simulink model "adaptive_dcmotor_2nd_hw"  (R2025b)
settings: Solver=FixedStepAuto  StartTime=0.0  StopTime=inf  FixedStep=0.08  RelTol=1e-3  EnableMultiTasking=on
libraries: arduinolib x3, arduinosensorlib x1
settings Model: Creator=Lenard  LastModifiedBy=Felix
settings SolverCC: AutoInsertRateTranBlk=on
settings OptimizationCC: EnhancedBackFolding=on  PassReuseOutputArgsAs=Individual arguments  ZeroExternalMemoryAtStartup=off  ZeroInternalMemoryAtStartup=off  MaxStackSize=64  OptimizeBlockOrder=speed  DifferentSizesBufferReuse=on  OptimizationCustomize=off  EfficientTunableParamExpr=on
settings DebuggingCC: ParameterTunabilityLossMsg=error
settings HardwareCC: ProdBitPerPointer=32.0  ProdBitPerSizeT=32.0  ProdBitPerPtrDiffT=32.0  ProdLargestAtomicInteger=Long  ProdLargestAtomicFloat=Double  ProdWordSize=32.0  ProdHWDeviceType=ARM Compatible->ARM Cortex
settings SFSimCC: MATLABDynamicMemAlloc=off
settings RTWCC: SystemTargetFile=ert.tlc  HardwareBoard=ESP32-WROOM (Arduino Compatible)  TLCOptions="-aInlineSetEventsForThisBaseRateFcn=TLC_FALSE -aSuppressMultiTaskScheduler=TLC_FALSE  -aRateBasedStepFcn=0"  TemplateMakefile=ert_default_tmf  Toolchain=ESP32  BuildConfiguration=Faster Runs  Description=Embedded Coder
settings CodeAppCC: ForceParamTrailComments=on  IgnoreCustomStorageClasses=off  OperatorAnnotations=on  SimulinkDataObjDesc=on  SFDataObjDesc=on  InsertBlockDesc=on
settings ERTTargetCC: ExtModeTransport=3.0  ExtModeStaticAlloc=on  ExtModeAutomaticAllocSize=off  ExtModeStaticAllocSize=65536.0  ExtModeMexFile=ext_xcp  ExtModeIntrfLevel=Level2 - Open  InlinedParameterPlacement=Hierarchical  SupportContinuousTime=on  SupportVariableSizeSignals=on

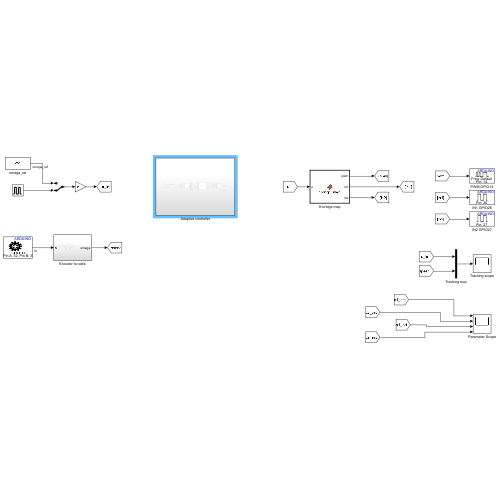
[thumbnail: Simulink's stored preview of the top-level diagram]
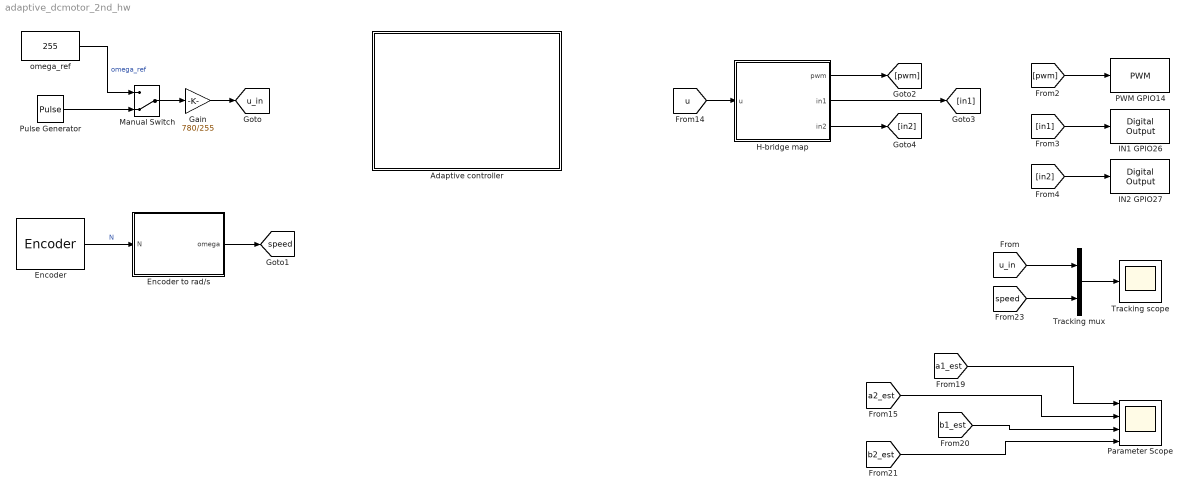
== system adaptive_dcmotor_2nd_hw ==
  Adaptive controller : Subsystem
  Encoder : arduinosensorlib/Encoder  InputA=32  InputB=33  Mode=No reset  SampleTime=0.08
  Encoder to rad/s : Subsystem
  Gain : Gain  Gain=780/255
  H-bridge map : MATLAB Function  TreatAsAtomicUnit=on
  IN1 GPIO26 : arduinolib/Digital Output  pinNumber=26  Direction=output  blockPlatform=arduino
  IN2 GPIO27 : arduinolib/Digital Output  pinNumber=27  Direction=output  blockPlatform=arduino
  Manual Switch : ManualSwitch  CurrentSetting=0
  PWM GPIO14 : arduinolib/PWM  pinNumber=14  frequencyType=Default  desiredFrequency=490.2  achievableFrequency=490.2
  Parameter Scope : Scope  NumInputPorts=4
      settings: ActiveDisplayYMinimum=-1590.0375907934126  ActiveDisplayYMaximum=2454.7527089363357
  Pulse Generator : DiscretePulseGenerator  PulseType=Time based  Amplitude=255  Period=8  PulseWidth=50  VectorParams1D=off
  Tracking mux : Mux  Inputs=2
  Tracking scope : Scope
      settings: ActiveDisplayYMinimum=-11603.301483749512  ActiveDisplayYMaximum=9185.7875106822521  DataLoggingVariableName=step
  omega_ref : Constant  Value=255  SampleTime=0.08
  tag scope: speed=global, u_in=global
  wires:
  Encoder/1 -> Encoder to rad/s/1(N)  "N"
  Pulse Generator/1 -> Manual Switch/2
  Gain/1 -> [u_in]
  Manual Switch/1 -> Gain/1
  omega_ref/1 -> Manual Switch/1  "omega_ref"
  Encoder to rad/s/1(omega) -> [speed]
  [pwm] -> PWM GPIO14/1
  [in1] -> IN1 GPIO26/1
  [in2] -> IN2 GPIO27/1
  H-bridge map/1(pwm) -> [pwm]
  H-bridge map/2(in1) -> [in1]
  H-bridge map/3(in2) -> [in2]
  [u] -> H-bridge map/1(u)
  Tracking mux/1 -> Tracking scope/1
  [u_in] -> Tracking mux/1
  [speed] -> Tracking mux/2
  [a2_est] -> Parameter Scope/2
  [b2_est] -> Parameter Scope/4
  [a1_est] -> Parameter Scope/1
  [b1_est] -> Parameter Scope/3

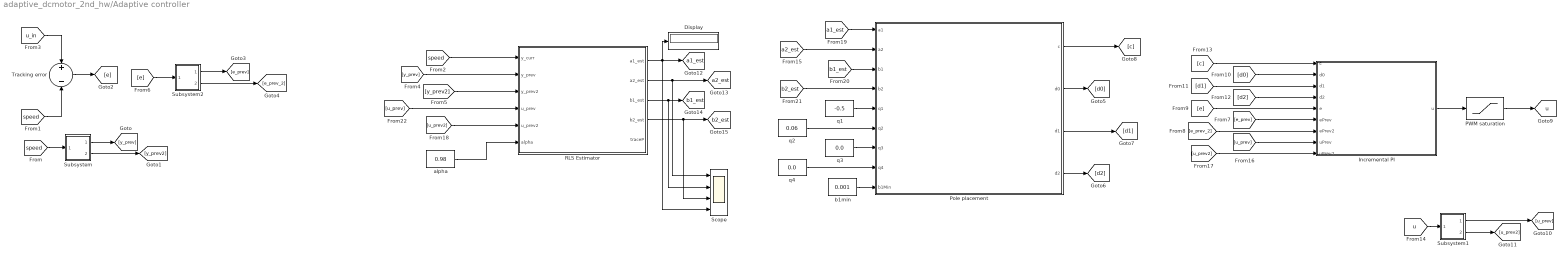
== system adaptive_dcmotor_2nd_hw/Adaptive controller ==
  Display : Display
  Incremental PI : MATLAB Function  TreatAsAtomicUnit=on
  PWM saturation : Saturate  UpperLimit=255  LowerLimit=0
  Pole placement : MATLAB Function  TreatAsAtomicUnit=on
  RLS Estimator : MATLAB Function  TreatAsAtomicUnit=on
  Scope : Scope  NumInputPorts=4
      settings: ActiveDisplayYMinimum=-1.9835538940406421  ActiveDisplayYMaximum=2.3467419345122842  DataLoggingVariableName=param
  Subsystem : Subsystem
  Subsystem1 : Subsystem
  Subsystem2 : Subsystem
  Tracking error : Sum  Inputs=+-
  alpha : Constant  Value=0.98
  b1min : Constant  Value=0.001
  q1 : Constant  Value=-0.5
  q2 : Constant  Value=0.06
  q3 : Constant  Value=0.0
  q4 : Constant  Value=0.0
  tag scope: a1_est=global, a2_est=global, b1_est=global, b2_est=global, u=global
  wires:
  alpha/1 -> RLS Estimator/6(alpha)
  Incremental PI/1(u) -> PWM saturation/1
  PWM saturation/1 -> [u]
  Pole placement/1(c) -> [c]
  q1/1 -> Pole placement/5(q1)
  q2/1 -> Pole placement/6(q2)
  q3/1 -> Pole placement/7(q3)
  q4/1 -> Pole placement/8(q4)
  b1min/1 -> Pole placement/9(b1Min)
  Subsystem1/1(Out1) -> [u_prev]
  Subsystem1/2(Out2) -> [u_prev2]
  [speed] -> Tracking error/2
  [speed] -> RLS Estimator/1(y_curr)
  [speed] -> Subsystem/1(In1)
  [u_in] -> Tracking error/1
  Subsystem/1(Out1) -> [y_prev]
  [y_prev] -> RLS Estimator/2(y_prev)
  Subsystem/2(Out2) -> [y_prev2]
  [y_prev2] -> RLS Estimator/3(y_prev2)
  Tracking error/1 -> [e]
  [e] -> Subsystem2/1(In1)
  Subsystem2/1(Out1) -> [e_prev]
  [e_prev] -> Incremental PI/6(ePrev)
  Subsystem2/2(Out2) -> [e_prev_2]
  [e_prev_2] -> Incremental PI/7(ePrev2)
  [e] -> Incremental PI/5(e)
  Pole placement/2(d0) -> [d0]
  Pole placement/3(d1) -> [d1]
  Pole placement/4(d2) -> [d2]
  [d0] -> Incremental PI/2(d0)
  [d1] -> Incremental PI/3(d1)
  [d2] -> Incremental PI/4(d2)
  [c] -> Incremental PI/1(c)
  [u] -> Subsystem1/1(In1)
  [u_prev] -> RLS Estimator/4(u_prev)
  [u_prev] -> Incremental PI/8(uPrev)
  [u_prev2] -> Incremental PI/9(uPrev2)
  [u_prev2] -> RLS Estimator/5(u_prev2)
  RLS Estimator/1(a1_est) -> Scope/4, Display/1, [a1_est]
  [a1_est] -> Pole placement/1(a1)
  RLS Estimator/2(a2_est) -> Scope/1, [a2_est]
  [a2_est] -> Pole placement/2(a2)
  RLS Estimator/3(b1_est) -> Scope/2, [b1_est]
  [b1_est] -> Pole placement/3(b1)
  RLS Estimator/4(b2_est) -> Scope/3, [b2_est]
  [b2_est] -> Pole placement/4(b2)

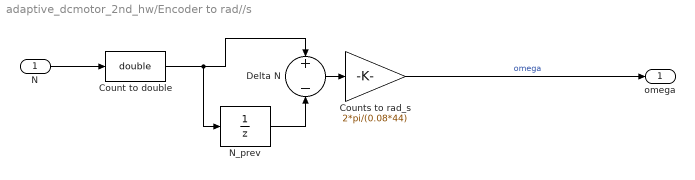
== system adaptive_dcmotor_2nd_hw/Encoder to rad//s ==
  N : Inport
  Count to double : DataTypeConversion  OutDataTypeStr=double  SaturateOnIntegerOverflow=off  RndMeth=Floor
  Counts to rad_s : Gain  Gain=2*pi/(0.08*44)
  Delta N : Sum  Inputs=+-
  N_prev : UnitDelay  SampleTime=0.08  HasFrameUpgradeWarning=on
  omega : Outport
  wires:
  N_prev/1 -> Delta N/2
  Count to double/1 -> N_prev/1, Delta N/1
  Delta N/1 -> Counts to rad_s/1
  Counts to rad_s/1 -> omega/1  "omega"
  N/1 -> Count to double/1

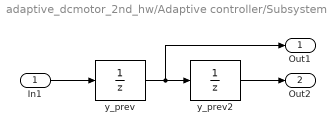
== system adaptive_dcmotor_2nd_hw/Adaptive controller/Subsystem ==
  In1 : Inport
  y_prev : UnitDelay  SampleTime=0.08  HasFrameUpgradeWarning=on
  y_prev2 : UnitDelay  SampleTime=0.08  HasFrameUpgradeWarning=on
  Out1 : Outport
  Out2 : Outport  Port=2
  wires:
  y_prev/1 -> Out1/1, y_prev2/1
  y_prev2/1 -> Out2/1
  In1/1 -> y_prev/1

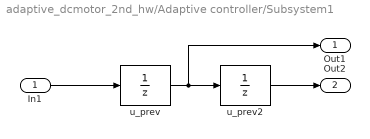
== system adaptive_dcmotor_2nd_hw/Adaptive controller/Subsystem1 ==
  In1 : Inport
  u_prev : UnitDelay  SampleTime=0.08  HasFrameUpgradeWarning=on
  u_prev2 : UnitDelay  SampleTime=0.08  HasFrameUpgradeWarning=on
  Out1 : Outport
  Out2 : Outport  Port=2
  wires:
  In1/1 -> u_prev/1
  u_prev/1 -> Out1/1, u_prev2/1
  u_prev2/1 -> Out2/1

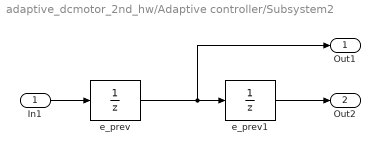
== system adaptive_dcmotor_2nd_hw/Adaptive controller/Subsystem2 ==
  In1 : Inport
  e_prev : UnitDelay  SampleTime=0.08  HasFrameUpgradeWarning=on
  e_prev1 : UnitDelay  SampleTime=0.08  HasFrameUpgradeWarning=on
  Out1 : Outport
  Out2 : Outport  Port=2
  wires:
  e_prev/1 -> Out1/1, e_prev1/1
  e_prev1/1 -> Out2/1
  In1/1 -> e_prev/1

== matlab function adaptive_dcmotor_2nd_hw/Adaptive controller/Pole placement ==
  data: c output; a1 input; a2 input; b1 input; b2 input; q1 input; q2 input; q3 input; q4 input; d0 output; b1Min input; d1 output; d2 output
function [c, d0, d1, d2] = pole_placement(a1, a2, b1, b2, q1, q2, q3, q4, b1Min)
    %#codegen
    persistent cHold d0Hold d1Hold d2Hold
    
    if isempty(cHold)
        % Defaults to a standard integrator logic (c = -1)
        cHold = -1.0; 
        d0Hold = 1.5; 
        d1Hold = -1.0;
        d2Hold = 0.0;
    end
    
    % GUARD: Ensure plant parameters are large enough to avoid singular matrices
    if abs(b1) > b1Min || abs(b2) > b1Min
        
        % 4x4 Sylvester Matrix for A(z)S(z) + B(z)R(z)
        M = [ 1,         b1,  0,  0;
              a1 - 1,    b2,  b1, 0;
              a2 - a1,   0,   b2, b1;
             -a2,        0,   0,  b2 ];
             
        % Desired closed-loop polynomial Q(z) constants
        Y = [ q1 - a1;
              q2 - a2 + 1;
              q3 + a1;
              q4 + a2 ];
              
        % Solve for X = [c; d0; d1; d2]
        X = M \ Y;
        
        % GUARD 2: Check for valid mathematical solution to avoid Simulink crashing
        if all(isfinite(X))
            cHold  = X(1);
            d0Hold = X(2);
            d1Hold = X(3);
            d2Hold = X(4);
        end
    end
    
    c  = cHold;
    d0 = d0Hold;
    d1 = d1Hold;
    d2 = d2Hold;
end

== matlab function adaptive_dcmotor_2nd_hw/Adaptive controller/RLS Estimator ==
  data: y_curr input; a1_est output; y_prev input; y_prev2 input; u_prev input; u_prev2 input; alpha input; a2_est output; b1_est output; b2_est output; traceP output
function [a1_est, a2_est, b1_est, b2_est, traceP] = rls_estimator(y_curr, y_prev, y_prev2, u_prev, u_prev2, alpha)     
    persistent P xe                                                            
    
    if isempty(P)                                                              
        P = 10.0 * eye(4);                                                   
        xe = [-0.5; 0.0; 1.0; 0.0];                                                      
    end    
    
    C = [-y_prev, -y_prev2, u_prev, u_prev2];    
    
    if (C * C') > 1e-6                                                         
        den = C * P * C' + alpha;                                              
        L = (P * C') / den;                                                    
        xe = xe + L * (y_curr - C * xe);                                       
        P = (eye(4) - L * C) * P / alpha;                                      
        P = 0.5 * (P + P');                                                    
    end  
    
    a1_est = xe(1);                                                            
    a2_est = xe(2);    
    b1_est = xe(3);
    b2_est = xe(4);
    traceP = trace(P);                                                  
end

== matlab function adaptive_dcmotor_2nd_hw/Adaptive controller/Incremental PI ==
  data: c input; d0 input; u output; d1 input; d2 input; e input; ePrev input; ePrev2 input; uPrev input; uPrev2 input
function u = adaptive_controller(c, d0, d1, d2, e, ePrev, ePrev2, uPrev, uPrev2)
    %#codegen
    % Implements the control law: S(z)U(z) = R(z)E(z)
    % S(z) = 1 + c*z^-1 - (1+c)*z^-2  (Guarantees integral action sum is 0)
    % R(z) = d0 + d1*z^-1 + d2*z^-2
    
    % Apply the discrete control law with the new degree of freedom
    u = -c * uPrev + (1 + c) * uPrev2 + d0 * e + d1 * ePrev + d2 * ePrev2;
end

== matlab function adaptive_dcmotor_2nd_hw/H-bridge map ==
  data: u input; pwm output; in1 output; in2 output
function [pwm,in1,in2] = hbridge_map(u)                    
                                                          %#codegen                                                  
                                                          % |u| -> PWM duty (0..255), sign(u) -> L298N direction pins
                                                          pwm = abs(u);                                              
                                                          if u >= 0                                                  
                                                              in1 = 1; in2 = 0;                                      
                                                          else                                                       
                                                              in1 = 0; in2 = 1;                                      
                                                          end                                                        
                                                          end
